simulink model "PID_CONTROL_CASE"  (R2023a)
settings: Solver=VariableStepAuto  StartTime=0.0  StopTime=5  RelTol=1e-3
values from neighbouring files (symbols this model uses):
  A = 13.13    [SIMULATION_PARAMETERS.m]
  b = 0.944    [SIMULATION_PARAMETERS.m]
  C_m = 0.8    [SIMULATION_PARAMETERS.m]
  C_panels = 0.05    [SIMULATION_PARAMETERS.m]
  J_panels = 778.58256    [SIMULATION_PARAMETERS.m]
  K_t = 0.02271    [SIMULATION_PARAMETERS.m]
  L_motor = 1.066e-3    (= 0.001066)    [SIMULATION_PARAMETERS.m]
  r_large = 20    [SIMULATION_PARAMETERS.m]
  R_motor = 0.044    [SIMULATION_PARAMETERS.m]
  r_small = 1    [SIMULATION_PARAMETERS.m]
  rho = 1.225    [SIMULATION_PARAMETERS.m]
  Theta_max = 2*pi    (= 6.28318530718)    [SIMULATION_PARAMETERS.m]
  V_max = 12    [SIMULATION_PARAMETERS.m]
libraries: slpidlib x1
settings Model: Creator=ssphe  LastModifiedBy=ssphe

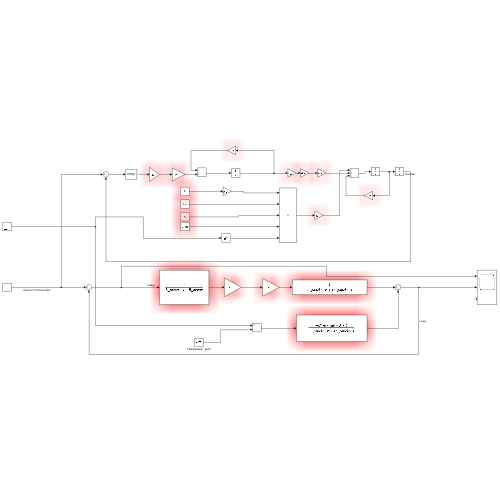
[thumbnail: Simulink's stored preview of the top-level diagram]
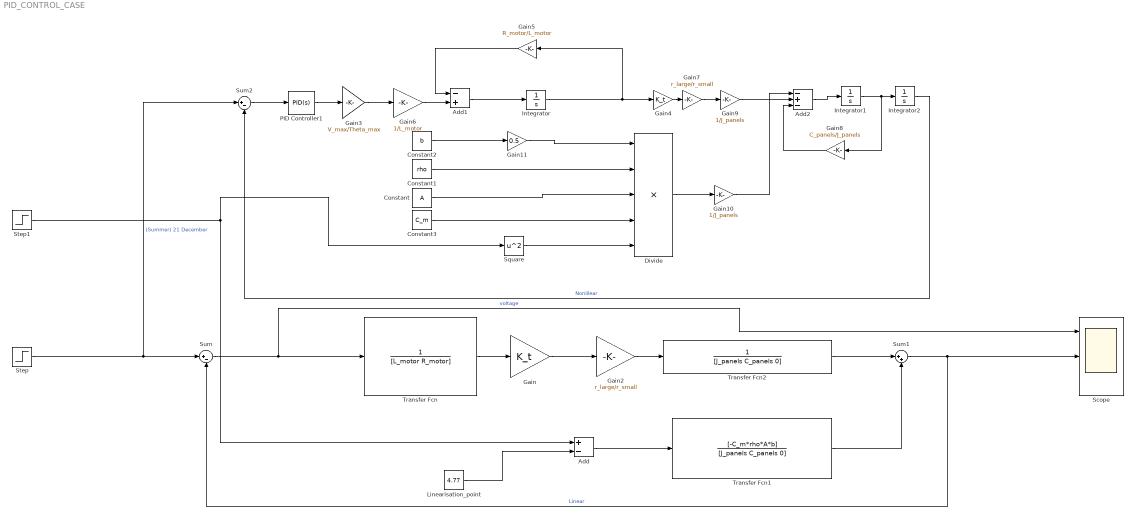
== system PID_CONTROL_CASE ==
  Add : Sum  Inputs=+-
  Add1 : Sum  Inputs=-+
  Add2 : Sum  Inputs=-+-
  Constant : Constant  Value=A
  Constant1 : Constant  Value=rho
  Constant2 : Constant  Value=b
  Constant3 : Constant  Value=C_m
  Divide : Product  Inputs=*****
  Gain : Gain  Gain=K_t
  Gain10 : Gain  Gain=1/J_panels
  Gain11 : Gain  Gain=0.5
  Gain2 : Gain  Gain=r_large/r_small
  Gain3 : Gain  Gain=V_max/Theta_max
  Gain4 : Gain  Gain=K_t
  Gain5 : Gain  Gain=R_motor/L_motor
  Gain6 : Gain  Gain=1/L_motor
  Gain7 : Gain  Gain=r_large/r_small
  Gain8 : Gain  Gain=C_panels/J_panels
  Gain9 : Gain  Gain=1/J_panels
  Integrator : Integrator
  Integrator1 : Integrator
  Integrator2 : Integrator
  Linearisation_point : Constant  Value=4.77
  PID Controller1 : slpidlib/PID Controller  Controller=PID  Form=Parallel  TimeDomain=Continuous-time  UseExternalTs=off  SampleTime=-1  IntegratorMethod=Forward Euler  FilterMethod=Forward Euler  ControllerParametersSource=internal  P=608.97763487089  I=124.228683688285  UseKiTs=off  D=458.770088343086  N=1288.11199821961  UseFilter=on  TunerSelectOption=Transfer Function Based (PID Tuner App)  InitialConditionSource=internal  InitialConditionForIntegrator=0  InitialConditionForFilter=0  DifferentiatorICPrevScaledInput=0  ExternalReset=none  TrackingMode=off  Kt=1  LimitOutput=off  SatLimitsSource=internal  UpperSaturationLimit=inf  LowerSaturationLimit=-inf  LinearizeAsGain=on  AntiWindupMode=none  Kb=1  LimitIntegrator=off  UpperIntegratorSaturationLimit=inf  LowerIntegratorSaturationLimit=-inf  POutMin=[]  POutMax=[]  IOutMin=[]  IOutMax=[]  DOutMin=[]  DOutMax=[]  NOutMin=[]  NOutMax=[]  SumOutMin=[]  SumOutMax=[]  SaturationOutMin=[]  SaturationOutMax=[]  PParamMin=[]  PParamMax=[]  IParamMin=[]  IParamMax=[]  DParamMin=[]  DParamMax=[]  NParamMin=[]  NParamMax=[]  KbParamMin=[]  KbParamMax=[]  KtParamMin=[]  KtParamMax=[]  KbOutMin=[]  KbOutMax=[]  KtOutMin=[]  KtOutMax=[]  IntegratorOutMin=[]  IntegratorOutMax=[]  FilterOutMin=[]  FilterOutMax=[]  SumI1OutMin=[]  SumI1OutMax=[]  SumI2OutMin=[]  SumI2OutMax=[]  SumI3OutMin=[]  SumI3OutMax=[]  SumI4OutMin=[]  SumI4OutMax=[]  SumDOutMin=[]  SumDOutMax=[]  DifferentiatorOutMin=[]  DifferentiatorOutMax=[]  FilterDiffOutCoefMin=[]  FilterDiffOutCoefMax=[]  ReciprocalOutMin=[]  ReciprocalOutMax=[]  SumDenOutMin=[]  SumDenOutMax=[]  SumNumOutMin=[]  SumNumOutMax=[]  DivideOutMin=[]  DivideOutMax=[]  UdiffTsProdOutMin=[]  UdiffTsProdOutMax=[]  NTsProdOutMin=[]  NTsProdOutMax=[]  UintegralTsProdOutMin=[]  UintegralTsProdOutMax=[]  UngainTsProdOutMin=[]  UngainTsProdOutMax=[]  ClampingZeroOutDataTypeStr=Inherit: Inherit via back propagation  ClampingZeroOutMin=[]  ClampingZeroOutMax=[]  FilterDenConstantOutDataTypeStr=Inherit: Inherit via back propagation  FilterDenConstantOutMin=[]  FilterDenConstantOutMax=[]  PCopyOutDataTypeStr=Inherit: Inherit via back propagation  PCopyOutMin=[]  PCopyOutMax=[]  NCopyOutDataTypeStr=Inherit: Inherit via back propagation  NCopyOutMin=[]  NCopyOutMax=[]  IntegratorContinuousStateAttributes=''  IntegratorStateMustResolveToSignalObject=off  IntegratorRTWStateStorageClass=Auto  FilterContinuousStateAttributes=''  FilterStateMustResolveToSignalObject=off  FilterRTWStateStorageClass=Auto  ParallelPVariant=InternalParameters  IdealPVariant=Disabled  IVariant=InternalParameters  DVariant=InternalParameters  IntegratorVariant=Continuous  SatVariant=Disabled  AWVariant=Passthrough  PCopyVariant=Disabled  TRVariant=Disabled  FdbkBlocksVariant=Forward  IdealPFdbkVariant=Disabled  SatFdbkVariant=Disabled  DerivativeFilterVariant=ContFilter  NVariant=InternalParameters  NCopyVariant=Disabled  FilterICVariant=InternalICsFilter  IntegratorICVariant=InternalICs  ExternalResetVariant=Disabled  TRSumVariant=Passthrough  SumFdbkVariant=Disabled  SumVariant=Sum_PID  TsampFilterVariant=InternalTs  TsampNgainVariant=Passthrough  TsampIntegralVariant=Disabled_SignalSpec  ExternalSaturationOutDataTypeStr=Inherit: Same as second input
  Scope : Scope  NumInputPorts=3
  Square : Math  Operator=square
  Step : Step  Time=0  SampleTime=0
  Step1 : Step  Time=0  After=5  SampleTime=0
  Sum : Sum  Inputs=|+-
  Sum1 : Sum  Inputs=|++
  Sum2 : Sum  Inputs=|+-
  Transfer Fcn : TransferFcn  Denominator=[L_motor R_motor]
  Transfer Fcn1 : TransferFcn  Numerator=[-C_m*rho*A*b]  Denominator=[J_panels C_panels 0]
  Transfer Fcn2 : TransferFcn  Denominator=[J_panels C_panels 0]
  wires:
  Sum/1 -> Scope/1, Transfer Fcn/1  "voltage"
  Transfer Fcn/1 -> Gain/1
  Gain/1 -> Gain2/1
  Gain2/1 -> Transfer Fcn2/1
  Add/1 -> Transfer Fcn1/1
  Linearisation_point/1 -> Add/2
  Transfer Fcn2/1 -> Sum1/1
  Transfer Fcn1/1 -> Sum1/2
  Sum1/1 -> Sum/2, Scope/2  "Linear"
  Gain9/1 -> Add2/2
  Gain8/1 -> Add2/3
  Sum2/1 -> PID Controller1/1
  Gain6/1 -> Add1/2
  Constant1/1 -> Divide/2
  Integrator1/1 -> Gain8/1, Integrator2/1
  Add2/1 -> Integrator1/1
  Gain4/1 -> Gain7/1
  Square/1 -> Divide/5
  Gain7/1 -> Gain9/1
  Constant3/1 -> Divide/4
  Gain10/1 -> Add2/1
  Integrator/1 -> Gain5/1, Gain4/1
  Divide/1 -> Gain10/1
  Constant/1 -> Divide/3
  Step1/1 -> Square/1, Add/1
  Integrator2/1 -> Sum2/2  "Nonlilear"
  Add1/1 -> Integrator/1
  Gain3/1 -> Gain6/1
  Constant2/1 -> Gain11/1
  Gain5/1 -> Add1/1
  Step/1 -> Sum2/1, Sum/1  "(Summer) 21 December"
  Gain11/1 -> Divide/1
  PID Controller1/1 -> Gain3/1
